simulink model "optionAModel1"  (R2019a)
settings: Solver=VariableStepAuto  StartTime=0.0  StopTime=10.0  RelTol=1e-3
model mask{optionB=optionB}
model workspace (MAT data in the model file):
  A = 1
  optionB = 1
settings Model: ParameterArgumentNames=optionB  OrderedModelArguments=off  Creator=jnicholson  LastModifiedBy=jnicholson

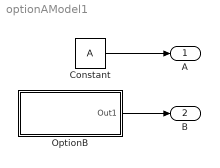
== system optionAModel1 ==
  Constant : Constant  Value=A
  OptionB : Subsystem  VariantControlMode=Label  Variant=on  LabelModeActiveChoice=ModelB1
  A : Outport
  B : Outport  Port=2
  wires:
  Constant/1 -> A/1
  OptionB/1(Out1) -> B/1

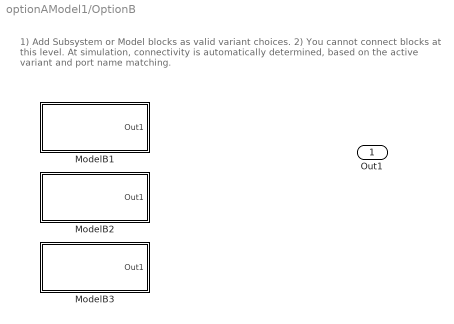
== system optionAModel1/OptionB ==
  note: 1) Add Subsystem or Model blocks as valid variant choices.
      | 2) You cannot connect blocks at this level. At simulation, connectivity is automatically
      | determined, based on the active variant and port name matching.
  ModelB1 : Subsystem  VariantControl=ModelB1
  ModelB2 : Subsystem  VariantControl=ModelB2
  ModelB3 : Subsystem  VariantControl=ModelB3
  Out1 : Outport

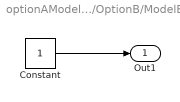
== system optionAModel1/OptionB/ModelB1 ==
  Constant : Constant
  Out1 : Outport
  wires:
  Constant/1 -> Out1/1

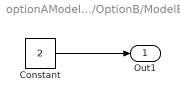
== system optionAModel1/OptionB/ModelB2 ==
  Constant : Constant  Value=2
  Out1 : Outport
  wires:
  Constant/1 -> Out1/1

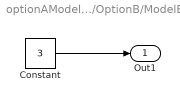
== system optionAModel1/OptionB/ModelB3 ==
  Constant : Constant  Value=3
  Out1 : Outport
  wires:
  Constant/1 -> Out1/1
